simulink model "DoublePendulum_withnoise"  (R2021b)
settings: Solver=VariableStepAuto  StartTime=0.0  StopTime=30  MaxStep=1e-3  RelTol=1e-3
PreLoadFcn:
  | initDoublePendulum
InitFcn:
  | initDoublePendulumParameters
  | initPendelumControl3x4
undefined symbols (not defined in the file): cartMass, cartPosLimits, controllerForDoublePendulum, initFeedback, pendulumMass, smiData, Ts, X, Y, Z
libraries: sm_lib x34, nesl_utility x12, simulink x7, sharedTrackingLibrary x2, cstblocks x2, fl_ps_legacy_lib x2, limitVelocityByPositionLimits x2
(part 2 of 2)

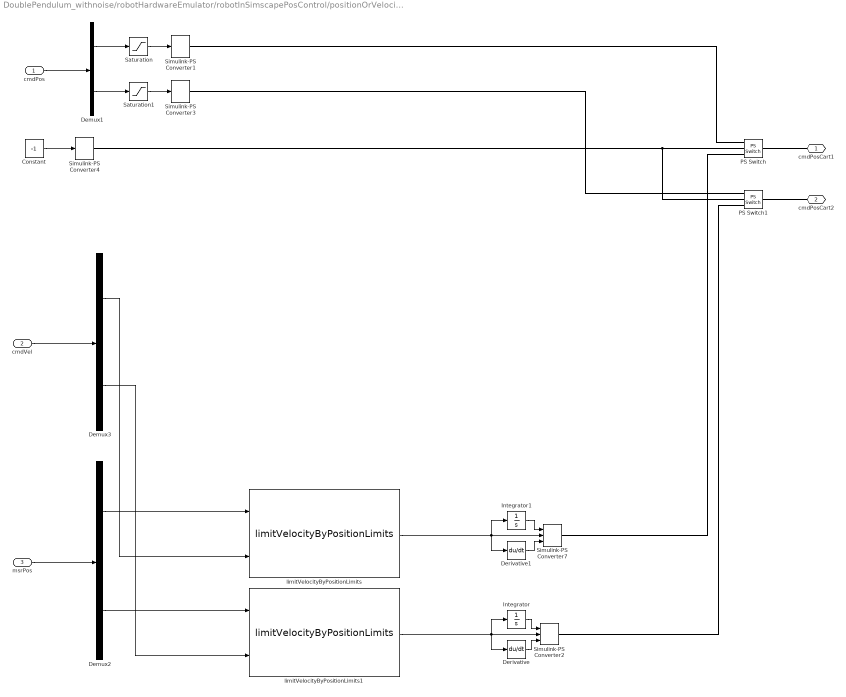
== system DoublePendulum_withnoise/robotHardwareEmulator/robotInSimscapePosControl/positionOrVelocityControlSelector ==
  cmdPos : Inport
  cmdVel : Inport  Port=2
  msrPos : Inport  Port=3
  Constant : Constant  Value=-1
  Demux1 : Demux  Outputs=2
  Demux2 : Demux  Outputs=2
  Demux3 : Demux  Outputs=2
  Derivative : Derivative
  Derivative1 : Derivative
  Integrator : Integrator  InitialCondition=initFeedback.cartPos(2)
  Integrator1 : Integrator  InitialCondition=initFeedback.cartPos(1)
  PS Switch : fl_ps_legacy_lib/Legacy Physical Signals/Nonlinear Operators/PS Switch  Threshold=0
      settings: SourceProductBaseCode=SS  InternalSimscapePortConfiguration="{\"Bottom\":[],\"Left\":[{\"id\":\"I1\",\"label\":\"\",\"type\":\"input\"},{\"id\":\"I2\",\"label\":\"\",\"type\":\"input\"},{\"id\":\"I3\",\"label\":\"\",\"type\":\"input\"}],\"Right\":[{\"id\":\"O\",\"label\":\"\",\"type\":\"output\"}],\"Top\":[]}"
  PS Switch1 : fl_ps_legacy_lib/Legacy Physical Signals/Nonlinear Operators/PS Switch  Threshold=0
      settings: SourceProductBaseCode=SS  InternalSimscapePortConfiguration="{\"Bottom\":[],\"Left\":[{\"id\":\"I1\",\"label\":\"\",\"type\":\"input\"},{\"id\":\"I2\",\"label\":\"\",\"type\":\"input\"},{\"id\":\"I3\",\"label\":\"\",\"type\":\"input\"}],\"Right\":[{\"id\":\"O\",\"label\":\"\",\"type\":\"output\"}],\"Top\":[]}"
  Saturation : Saturate  UpperLimit=cartPosLimits(2)  LowerLimit=cartPosLimits(1)
  Saturation1 : Saturate  UpperLimit=cartPosLimits(2)  LowerLimit=cartPosLimits(1)
  Simulink-PS Converter1 : nesl_utility/Simulink-PS Converter  PhysicalDomain=network_engine_domain  SubClassName=ps_input  LeftPortType=input  RightPortType=output  PseudoPeriodic=off  Frequencies=[]  NoiseDistribution=none  NoiseParameters=[]  Unit=m  AffineConversion=off  FilteringAndDerivatives=filter  SimscapeFilterOrder=2  InputFilterTimeConstant=0.001  UdotUserProvided=0
      settings: SourceProductBaseCode=PW,SS
  Simulink-PS Converter2 : nesl_utility/Simulink-PS Converter  PhysicalDomain=network_engine_domain  SubClassName=ps_input  LeftPortType=input  RightPortType=output  PseudoPeriodic=off  Frequencies=[]  NoiseDistribution=none  NoiseParameters=[]  Unit=m  AffineConversion=off  FilteringAndDerivatives=provide  SimscapeFilterOrder=2  InputFilterTimeConstant=0.001  UdotUserProvided=2
      settings: SourceProductBaseCode=PW,SS
  Simulink-PS Converter3 : nesl_utility/Simulink-PS Converter  PhysicalDomain=network_engine_domain  SubClassName=ps_input  LeftPortType=input  RightPortType=output  PseudoPeriodic=off  Frequencies=[]  NoiseDistribution=none  NoiseParameters=[]  Unit=m  AffineConversion=off  FilteringAndDerivatives=filter  SimscapeFilterOrder=2  InputFilterTimeConstant=0.001  UdotUserProvided=0
      settings: SourceProductBaseCode=PW,SS
  Simulink-PS Converter4 : nesl_utility/Simulink-PS Converter  PhysicalDomain=network_engine_domain  SubClassName=ps_input  LeftPortType=input  RightPortType=output  PseudoPeriodic=off  Frequencies=[]  NoiseDistribution=none  NoiseParameters=[]  Unit=m  AffineConversion=off  FilteringAndDerivatives=filter  SimscapeFilterOrder=2  InputFilterTimeConstant=0.001  UdotUserProvided=0
      settings: SourceProductBaseCode=PW,SS
  Simulink-PS Converter7 : nesl_utility/Simulink-PS Converter  PhysicalDomain=network_engine_domain  SubClassName=ps_input  LeftPortType=input  RightPortType=output  PseudoPeriodic=off  Frequencies=[]  NoiseDistribution=none  NoiseParameters=[]  Unit=m  AffineConversion=off  FilteringAndDerivatives=provide  SimscapeFilterOrder=1  InputFilterTimeConstant=0.001  UdotUserProvided=2
      settings: SourceProductBaseCode=PW,SS
  limitVelocityByPositionLimits : limitVelocityByPositionLimits/limitVelocityByPositionLimits  upperJointLimit=cartPosLimits(2)  lowerJointLimit=cartPosLimits(1)
  limitVelocityByPositionLimits1 : limitVelocityByPositionLimits/limitVelocityByPositionLimits  upperJointLimit=cartPosLimits(2)  lowerJointLimit=cartPosLimits(1)
  cmdPosCart1 : PMIOPort  Side=Right
  cmdPosCart2 : PMIOPort  Port=2  Side=Right
  wires:
  Derivative/1 -> Simulink-PS Converter2/3
  limitVelocityByPositionLimits1/1 -> Derivative/1, Integrator/1, Simulink-PS Converter2/2
  Demux3/2 -> limitVelocityByPositionLimits1/2
  cmdVel/1 -> Demux3/1
  Demux2/2 -> limitVelocityByPositionLimits1/1
  Demux2/1 -> limitVelocityByPositionLimits/1
  msrPos/1 -> Demux2/1
  Integrator1/1 -> Simulink-PS Converter7/1
  Demux3/1 -> limitVelocityByPositionLimits/2
  Derivative1/1 -> Simulink-PS Converter7/3
  limitVelocityByPositionLimits/1 -> Derivative1/1, Simulink-PS Converter7/2, Integrator1/1
  Integrator/1 -> Simulink-PS Converter2/1
  Demux1/2 -> Saturation1/1
  Saturation/1 -> Simulink-PS Converter1/1
  Saturation1/1 -> Simulink-PS Converter3/1
  Demux1/1 -> Saturation/1
  cmdPos/1 -> Demux1/1
  Constant/1 -> Simulink-PS Converter4/1
  connections:
  Simulink-PS Converter2/RConn1 -- PS Switch1/LConn3
  Simulink-PS Converter7/RConn1 -- PS Switch/LConn3
  PS Switch/LConn2 -- Simulink-PS Converter4/RConn1 -- PS Switch1/LConn2
  Simulink-PS Converter1/RConn1 -- PS Switch/LConn1
  PS Switch1/LConn1 -- Simulink-PS Converter3/RConn1
  cmdPosCart1/RConn1 -- PS Switch/RConn1
  cmdPosCart2/RConn1 -- PS Switch1/RConn1

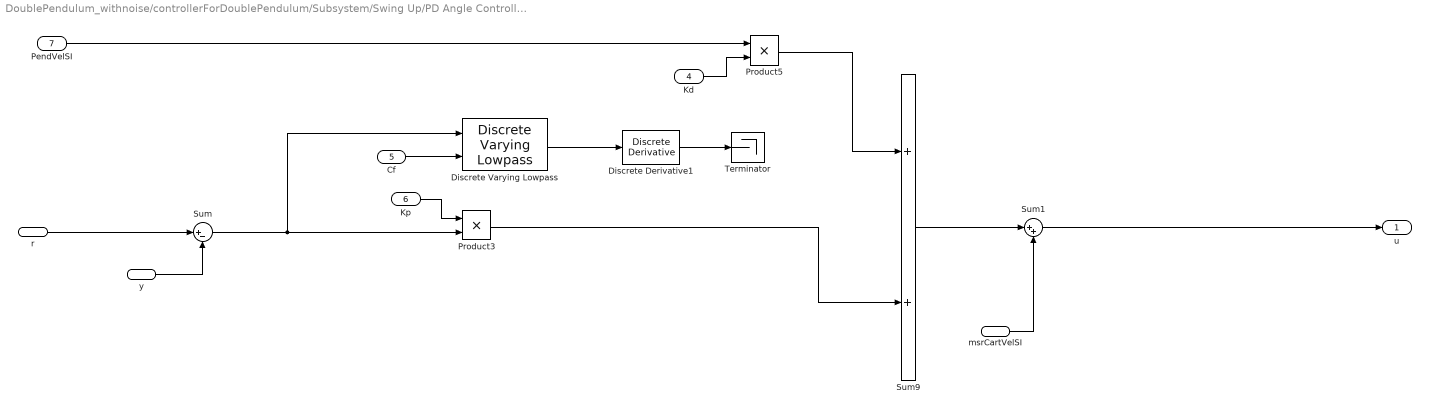
== system DoublePendulum_withnoise/controllerForDoublePendulum/Subsystem/Swing Up/PD Angle Controller ==
  msrCartVelSI : Inport
  r : Inport  Port=2
  y : Inport  Port=3
  Kd : Inport  Port=4
  Cf : Inport  Port=5
  Kp : Inport  Port=6
  PendVelSI : Inport  Port=7
  Discrete Derivative1 : simulink/Discrete/Discrete Derivative  gainval=1.0  ICPrevScaledInput=0.0  InputProcessing=Columns as channels (frame based)  OutMin=[]  OutMax=[]  OutDataType=fixdt(1, 16)  OutScaling=2^-10  DoSatur=off
  Discrete Varying Lowpass : cstblocks/Linear Parameter Varying/Discrete Varying Lowpass  N=1  w0=0  Ts=0.001
      settings: SourceProductBaseCode=CT
  Product3 : Product
  Product5 : Product
  Sum : Sum  Inputs=|+-
  Sum1 : Sum  Inputs=|++
  Sum9 : Sum
  Terminator : Terminator
  u : Outport
  wires:
  Kd/1 -> Product5/2
  Sum9/1 -> Sum1/1
  Kp/1 -> Product3/1
  Cf/1 -> Discrete Varying Lowpass/2
  Product5/1 -> Sum9/1
  Product3/1 -> Sum9/2
  Sum1/1 -> u/1
  y/1 -> Sum/2
  Sum/1 -> Discrete Varying Lowpass/1, Product3/2
  msrCartVelSI/1 -> Sum1/2
  Discrete Varying Lowpass/1 -> Discrete Derivative1/1
  Discrete Derivative1/1 -> Terminator/1
  PendVelSI/1 -> Product5/1
  r/1 -> Sum/1

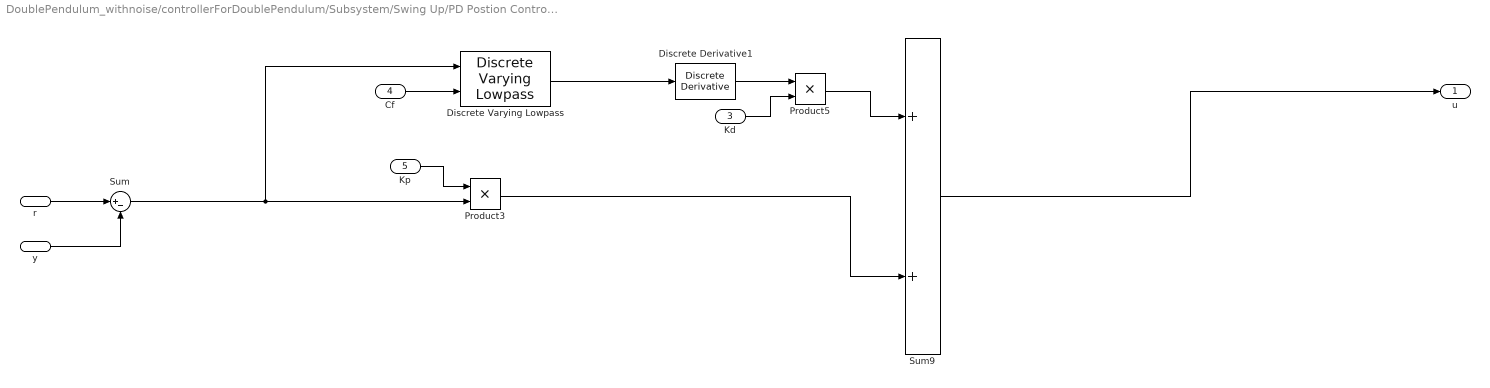
== system DoublePendulum_withnoise/controllerForDoublePendulum/Subsystem/Swing Up/PD Postion Controller ==
  r : Inport
  y : Inport  Port=2
  Kd : Inport  Port=3
  Cf : Inport  Port=4
  Kp : Inport  Port=5
  Discrete Derivative1 : simulink/Discrete/Discrete Derivative  gainval=1.0  ICPrevScaledInput=0.0  InputProcessing=Columns as channels (frame based)  OutMin=[]  OutMax=[]  OutDataType=fixdt(1, 16)  OutScaling=2^-10  DoSatur=off
  Discrete Varying Lowpass : cstblocks/Linear Parameter Varying/Discrete Varying Lowpass  N=1  w0=0  Ts=0.001
      settings: SourceProductBaseCode=CT
  Product3 : Product
  Product5 : Product
  Sum : Sum  Inputs=|+-
  Sum9 : Sum
  u : Outport
  wires:
  Sum/1 -> Product3/2, Discrete Varying Lowpass/1
  r/1 -> Sum/1
  y/1 -> Sum/2
  Cf/1 -> Discrete Varying Lowpass/2
  Discrete Derivative1/1 -> Product5/1
  Kp/1 -> Product3/1
  Kd/1 -> Product5/2
  Sum9/1 -> u/1
  Product5/1 -> Sum9/1
  Product3/1 -> Sum9/2
  Discrete Varying Lowpass/1 -> Discrete Derivative1/1

== matlab function DoublePendulum_withnoise/controllerForDoublePendulum/Subsystem/Wrap ==
  data: input input; y output
function y = fcn1(input)
    
persistent x
        
if isempty(x)
   x = 0;
end

if (input + x) > pi
    x = x -2*pi;
end

if (input + x) < -pi
    x = x + 2*pi;
end

y = input + x;

== matlab function DoublePendulum_withnoise/controllerForDoublePendulum/Subsystem/Swing Up/Angle in upper position ==
  data: input input; y output
function y  = fcn2(input)
    
if (input  >= 0)  
    y = -(input - pi);
else 
    y = -(input+pi);
end

== matlab function DoublePendulum_withnoise/controllerForDoublePendulum/Subsystem/Swing Up/Dwrap ==
  data: input input; y output
function y = fcn1(input)
    
persistent x
persistent inputOld
        
if isempty(x)
   x = 0;
   inputOld = input;
end

if (input < -0.5*pi) && (inputOld > 0.5*pi)
    x = x + 2*pi;
end

if (input > 0.5*pi) && (inputOld < -0.5*pi)
    x = x - 2*pi;
end

inputOld = input;

y = input + x;

== matlab function DoublePendulum_withnoise/controllerForDoublePendulum/Subsystem/Swing Up/Swing Up ==
  data: stateActual output; stateOld output; threshold input; PendlePos input; CartPos input; targetVelocityCart output; velocity input; posRight input; posLeft input; velocityAllowed input
function [stateActual, stateOld, targetVelocityCart] = fcn2(threshold, PendlePos,CartPos,velocity, posRight, posLeft, velocityAllowed)
    
persistent state
persistent stateLast

angleTreshold = pi- threshold*pi/180;
angleStart = threshold*pi/180;

if isempty(state) || isempty(stateLast)
   state = 0;
   stateLast = 0; 
end

if (abs(PendlePos) > angleTreshold) && (stateLast < 6)
    state = 6; 
end

if ~velocityAllowed
    state = 7; 
end 

stateOld = stateLast; 
stateActual = state; 
stateLast = state;

switch state   
    case 0
        targetVelocityCart = 0;
        if (abs(PendlePos) < angleStart)
            state = 1; 
        end       
    case 1
        if (CartPos <= posLeft) && (PendlePos >= 0)
            targetVelocityCart = velocity;
            state = 2;
        elseif (CartPos >= posRight) && (PendlePos <= 0)
            targetVelocityCart = -velocity;
            state = 3;
        elseif (posLeft < CartPos) && (CartPos < posRight)
            targetVelocityCart = velocity;
            state = 2;
        else
           targetVelocityCart = 0; 
        end           
    case 2
        if CartPos >= posRight
            targetVelocityCart = 0;
            state = 3;
        else 
            targetVelocityCart = velocity;
        end
    case 3
        if PendlePos <= 0
            targetVelocityCart = -velocity;
            state = 4;
        else 
            targetVelocityCart = 0;
        end
    case 4 
        if CartPos <= posLeft
            targetVelocityCart = 0;
            state = 5;
        else 
            targetVelocityCart = -velocity;
        end 
    case 5
        if PendlePos >= 0
            targetVelocityCart = velocity;
            state = 2;
        else 
            targetVelocityCart = 0;
        end
    case 6
        targetVelocityCart = 0;
        if (abs(PendlePos) < pi/2)
            state = 7; 
        end
    case 7
        targetVelocityCart = 0;
        if ~velocityAllowed
            state = 8; 
        end 
     case 8
        targetVelocityCart = 0;
        if velocityAllowed
            state = 0; 
        end 

    otherwise
        state = 0;
        targetVelocityCart = 0;
end
